simulink model "P5_1_SomeBlocks"  (R2025b)
settings: Solver=VariableStepAuto  StartTime=0.0  StopTime=10.0  MaxStep=1e-1  RelTol=1e-3
settings Model: Creator=tongx  LastModifiedBy=tongx

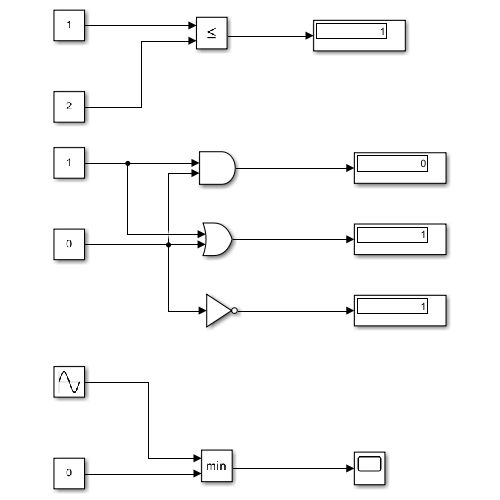
[thumbnail: Simulink's stored preview of the top-level diagram]
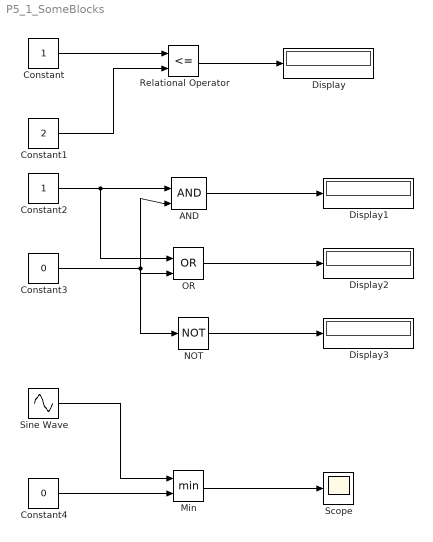
== system P5_1_SomeBlocks ==
  AND : Logic  IconShape=distinctive  AllPortsSameDT=off  OutDataTypeStr=boolean
  Constant : Constant
  Constant1 : Constant  Value=2
  Constant2 : Constant
  Constant3 : Constant  Value=0
  Constant4 : Constant  Value=0
  Display{,1..3} (4 alike) : Display
  Min : MinMax  Inputs=2
  NOT : Logic  Operator=NOT  IconShape=distinctive  AllPortsSameDT=off  OutDataTypeStr=boolean
  OR : Logic  Operator=OR  IconShape=distinctive  AllPortsSameDT=off  OutDataTypeStr=boolean
  Relational Operator : RelationalOperator  Operator=<=  OutDataTypeStr=boolean  RndMeth=Simplest  InputSameDT=off
  Scope : Scope
      settings: ActiveDisplayYMinimum=-1.1245203034216924  ActiveDisplayYMaximum=0.12494670038018803
  Sine Wave : Sin  Frequency=2  SampleTime=0
  wires:
  Constant/1 -> Relational Operator/1
  Constant1/1 -> Relational Operator/2
  Relational Operator/1 -> Display/1
  Constant2/1 -> OR/1, AND/1
  Constant3/1 -> AND/2, NOT/1, OR/2
  AND/1 -> Display1/1
  OR/1 -> Display2/1
  NOT/1 -> Display3/1
  Sine Wave/1 -> Min/1
  Constant4/1 -> Min/2
  Min/1 -> Scope/1
